simulink model "simu_4qc_transform"  (R2020a)
settings: Solver=FixedStepAuto  StartTime=0.0  StopTime=40  FixedStep=0.01  RelTol=1e-3
InitFcn:
  | init_conditions
values from neighbouring files (symbols this model uses):
  dgaina = 4e-5    (= 4e-05)    [init_conditions.m]
  dgainb = dgaina    (= 4e-05)    [init_conditions.m]
  fd0 = [0;0;m*g/4;0;0;m*g/4;0;0;m*g/4;0;0;m*g/4]    [init_conditions.m]
  g = 9.81    [init_conditions.m]
  IB = diag([IBxy, IBxy, IBz])    [init_conditions.m]
  igaina = 0e-5    (= 0)    [init_conditions.m]
  igainb = igaina    (= 0)    [init_conditions.m]
  Lh = 0.001    [init_conditions.m]
  Lw = 0.18    [init_conditions.m]
  m = (m_qc+0.006)*4 + m_main    (= 0.156)    [init_conditions.m]
  m_main = 0.012    [init_conditions.m]
  m_qc = 0.03    [init_conditions.m]
  np = [np1; np2; np3; np4; np5; ones(numpad,1)*np5(end,:)]    [init_conditions.m]
  pgaina = 1.5e-4    (= 0.00015)    [init_conditions.m]
  pgainb = pgaina    (= 0.00015)    [init_conditions.m]
  phi = zeros(num1+num2+num3+num4+num5+numpad, 1)    [init_conditions.m]
  psi = zeros(num1+num2+num3+num4+num5+numpad, 1)    [init_conditions.m]
  StepSize = 0.01    [init_conditions.m]
  the = [zeros(1,num1+num2), th, th(end) * ones(1, num4+num5+numpad)].'    [init_conditions.m]
undefined symbols (not defined in the file or in its folder): X, Y, Z
libraries: sm_lib x51, nesl_utility x26, simulink_extras x12, simulink x8, sharedtransform x1
(part 1 of 2)
settings Model: Creator=Paul  LastModifiedBy=Paul
settings DataIOCC: ReturnWorkspaceOutputs=off
settings DebuggingCC: ArithmeticOperatorsInVariantConditions=warning
settings SFSimCC: SimUseLocalCustomCode=off  CustomCodeUndefinedFunction=UseInterfaceOnly
settings RTWCC: RTWUseLocalCustomCode=off

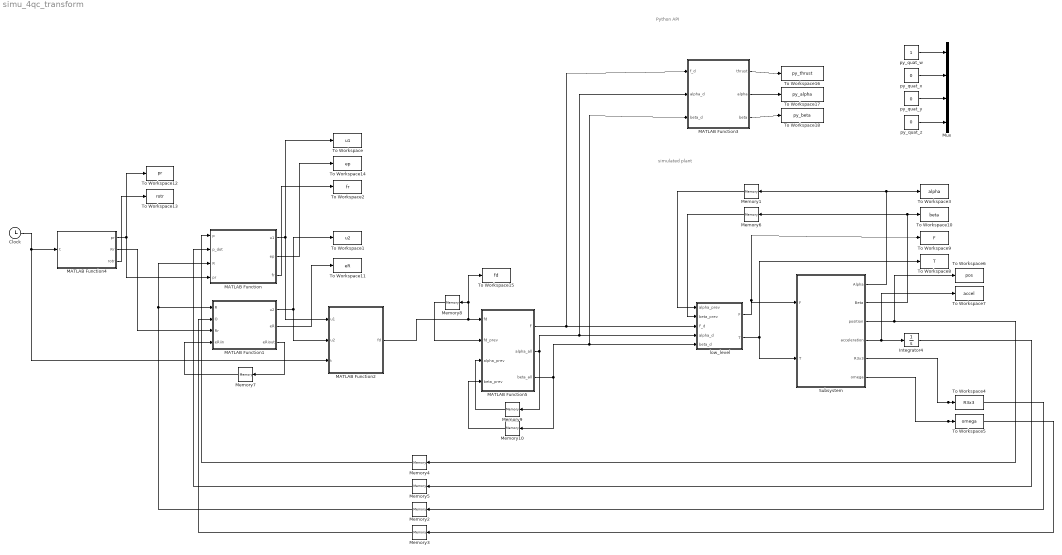
== system simu_4qc_transform ==
  note: Python API
  note: simulated plant
  Clock : Clock
  Integrator4 : Integrator  InitialCondition=[0;0;0]
  MATLAB Function : MATLAB Function  TreatAsAtomicUnit=on
  MATLAB Function1 : MATLAB Function  TreatAsAtomicUnit=on
  MATLAB Function2 : MATLAB Function  TreatAsAtomicUnit=on
  MATLAB Function3 : MATLAB Function  TreatAsAtomicUnit=on
  MATLAB Function4 : MATLAB Function  TreatAsAtomicUnit=on
  MATLAB Function5 : MATLAB Function  TreatAsAtomicUnit=on
  Memory{1,6,9..10} (4 alike) : Memory  InitialCondition=[0;0;0;0]
  Memory2 : Memory  InitialCondition=eye(3)
  Memory{3..5,7} (4 alike) : Memory  InitialCondition=[0;0;0]
  Memory8 : Memory  InitialCondition=fd0
  Mux : Mux
  Subsystem : Subsystem
  To Workspace : ToWorkspace  VariableName=u1  SaveFormat=Timeseries  SampleTime=-1
  To Workspace1 : ToWorkspace  VariableName=u2  SaveFormat=Timeseries  SampleTime=-1
  To Workspace10 : ToWorkspace  VariableName=beta  SaveFormat=Timeseries  SampleTime=-1
  To Workspace11 : ToWorkspace  VariableName=eR  SaveFormat=Timeseries  SampleTime=-1
  To Workspace12 : ToWorkspace  VariableName=pr  SaveFormat=Timeseries  SampleTime=-1
  To Workspace13 : ToWorkspace  VariableName=rotr  SaveFormat=Timeseries  SampleTime=-1
  To Workspace14 : ToWorkspace  VariableName=ep  SaveFormat=Timeseries  SampleTime=-1
  To Workspace15 : ToWorkspace  VariableName=fd  SaveFormat=Timeseries  SampleTime=-1
  To Workspace16 : ToWorkspace  VariableName=py_thrust  SampleTime=-1
      settings: Save2DSignal=2-D array (concatenate along first dimension)
  To Workspace17 : ToWorkspace  VariableName=py_alpha  SampleTime=-1
      settings: Save2DSignal=2-D array (concatenate along first dimension)
  To Workspace18 : ToWorkspace  VariableName=py_beta  SampleTime=-1
      settings: Save2DSignal=2-D array (concatenate along first dimension)
  To Workspace2 : ToWorkspace  VariableName=fr  SaveFormat=Timeseries  SampleTime=-1
  To Workspace3 : ToWorkspace  VariableName=alpha  SaveFormat=Timeseries  SampleTime=-1
  To Workspace4 : ToWorkspace  VariableName=R3x3  SaveFormat=Timeseries  SampleTime=-1
  To Workspace5 : ToWorkspace  VariableName=omega  SaveFormat=Timeseries  SampleTime=-1
  To Workspace6 : ToWorkspace  VariableName=pos  SaveFormat=Timeseries  SampleTime=-1
  To Workspace7 : ToWorkspace  VariableName=accel  SaveFormat=Timeseries  SampleTime=-1
  To Workspace8 : ToWorkspace  VariableName=T  SaveFormat=Timeseries  SampleTime=-1
  To Workspace9 : ToWorkspace  VariableName=F  SaveFormat=Timeseries  SampleTime=-1
  low_level : Subsystem
  py_quat_w : Constant
  py_quat_x : Constant  Value=0
  py_quat_y : Constant  Value=0
  py_quat_z : Constant  Value=0
  wires:
  MATLAB Function/1(u1) -> MATLAB Function2/1(u1), To Workspace/1
  MATLAB Function1/1(u2) -> MATLAB Function2/2(u2), To Workspace1/1
  Subsystem/5(R3x3) -> To Workspace4/1, Memory2/1
  Memory2/1 -> MATLAB Function1/1(R), MATLAB Function/3(R)
  Subsystem/6(omega) -> To Workspace5/1, Memory3/1
  Memory3/1 -> MATLAB Function1/2(O)
  Memory4/1 -> MATLAB Function/1(p)
  Memory5/1 -> MATLAB Function/2(p_dot)
  Subsystem/3(position) -> Memory4/1, To Workspace6/1
  Subsystem/4(acceleration) -> Integrator4/1, To Workspace7/1
  Integrator4/1 -> Memory5/1
  Clock/1 -> MATLAB Function2/3(t), MATLAB Function4/1(t)
  MATLAB Function4/1(pr) -> MATLAB Function/4(pr), To Workspace12/1
  MATLAB Function4/2(Rr) -> MATLAB Function1/3(Rr)
  MATLAB Function/3(fr) -> To Workspace2/1
  low_level/1(F) -> To Workspace9/1, Subsystem/1(F)
  low_level/2(T) -> To Workspace8/1, Subsystem/2(T)
  Subsystem/1(Alpha) -> To Workspace3/1, Memory1/1
  Subsystem/2(Beta) -> Memory6/1, To Workspace10/1
  Memory1/1 -> low_level/1(alpha_prev)
  Memory6/1 -> low_level/2(beta_prev)
  MATLAB Function1/2(eR) -> To Workspace11/1
  MATLAB Function4/3(rotr) -> To Workspace13/1
  MATLAB Function/2(ep) -> To Workspace14/1
  MATLAB Function1/3(eRiout) -> Memory7/1
  Memory7/1 -> MATLAB Function1/4(eRiin)
  Memory10/1 -> MATLAB Function5/4(beta_prev)
  Memory8/1 -> MATLAB Function5/2(fd_prev)
  MATLAB Function5/3(beta_all) -> MATLAB Function3/3(beta_d), low_level/5(beta_d), Memory10/1
  MATLAB Function5/2(alpha_all) -> MATLAB Function3/2(alpha_d), low_level/4(alpha_d), Memory9/1
  Memory9/1 -> MATLAB Function5/3(alpha_prev)
  MATLAB Function2/1(fd) -> To Workspace15/1, Memory8/1, MATLAB Function5/1(fd)
  MATLAB Function5/1(F) -> MATLAB Function3/1(f_d), low_level/3(F_d)
  MATLAB Function3/1(thrust) -> To Workspace16/1
  MATLAB Function3/2(alpha) -> To Workspace17/1
  MATLAB Function3/3(beta) -> To Workspace18/1
  py_quat_w/1 -> Mux/1
  py_quat_x/1 -> Mux/2
  py_quat_y/1 -> Mux/3
  py_quat_z/1 -> Mux/4

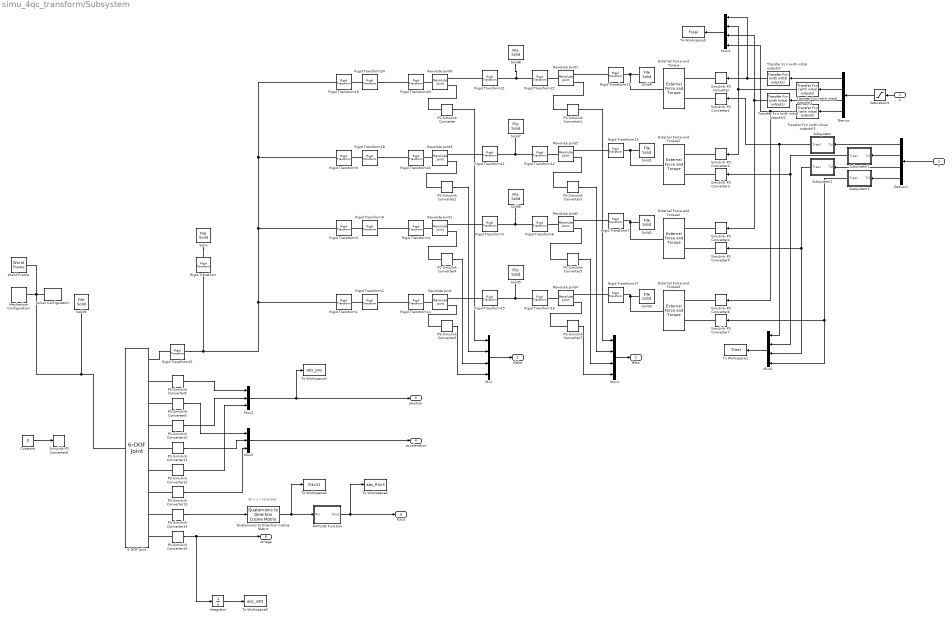
== system simu_4qc_transform/Subsystem ==
  note: all x y z reversed
  F : Inport
  T : Inport  Port=2
  6-DOF Joint : sm_lib/Joints/6-DOF Joint  JointMode=Normal  SenseConstraintForce=off  SenseConstraintForceX=off  SenseConstraintForceY=off  SenseConstraintForceZ=off  SenseConstraintTorque=off  SenseConstraintTorqueX=off  SenseConstraintTorqueY=off  SenseConstraintTorqueZ=off  SenseTotalForce=off  SenseTotalForceX=off  SenseTotalForceY=off  SenseTotalForceZ=off  SenseTotalTorque=off  SenseTotalTorqueX=off  SenseTotalTorqueY=off  SenseTotalTorqueZ=off  CompositeWrenchDir=FollowerOnBase  CompositeWrenchFrame=BaseFrame  PxEquilibriumPosition=0  PxEquilibriumPositionUnits=m  PxSpringStiffness=0  PxSpringStiffnessUnits=N/m  PxDampingCoefficient=0  PxDampingCoefficientUnits=N/(m/s)  PxTorqueActuationMode=NoTorque  PxMotionActuationMode=ComputedMotion  PxSensePosition=on  PxSenseVelocity=off  PxSenseAcceleration=on  PxSenseTorqueForce=off  PxSenseLowerLimitTorqueForce=off  PxSenseUpperLimitTorqueForce=off  PxLowerLimitSpecify=off  PxLowerLimitBound=-1  PxLowerLimitBoundUnits=m  PxLowerLimitStiffness=1e6  PxLowerLimitStiffnessUnits=N/m  PxLowerLimitDamping=1e3  PxLowerLimitDampingUnits=N/(m/s)  PxLowerLimitTransitionRegionWidth=1e-4  PxLowerLimitTransitionRegionWidthUnits=m  PxUpperLimitSpecify=off  PxUpperLimitBound=1  PxUpperLimitBoundUnits=m  PxUpperLimitStiffness=1e6  PxUpperLimitStiffnessUnits=N/m  PxUpperLimitDamping=1e3  PxUpperLimitDampingUnits=N/(m/s)  PxUpperLimitTransitionRegionWidth=1e-4  PxUpperLimitTransitionRegionWidthUnits=m  PxPositionTargetSpecify=off  PxPositionTargetPriority=High  PxPositionTargetValue=0  PxPositionTargetValueUnits=m  PxVelocityTargetSpecify=off  PxVelocityTargetPriority=High  PxVelocityTargetValue=0  PxVelocityTargetValueUnits=m/s  PyEquilibriumPosition=0  PyEquilibriumPositionUnits=m  PySpringStiffness=0  PySpringStiffnessUnits=N/m  PyDampingCoefficient=0  PyDampingCoefficientUnits=N/(m/s)  PyTorqueActuationMode=NoTorque  PyMotionActuationMode=ComputedMotion  PySensePosition=on  PySenseVelocity=off  PySenseAcceleration=on  PySenseTorqueForce=off  PySenseLowerLimitTorqueForce=off  PySenseUpperLimitTorqueForce=off  PyLowerLimitSpecify=off  PyLowerLimitBound=-1  PyLowerLimitBoundUnits=m  PyLowerLimitStiffness=1e6  PyLowerLimitStiffnessUnits=N/m  PyLowerLimitDamping=1e3  PyLowerLimitDampingUnits=N/(m/s)  PyLowerLimitTransitionRegionWidth=1e-4  PyLowerLimitTransitionRegionWidthUnits=m  PyUpperLimitSpecify=off  PyUpperLimitBound=1  PyUpperLimitBoundUnits=m  PyUpperLimitStiffness=1e6  PyUpperLimitStiffnessUnits=N/m  PyUpperLimitDamping=1e3  PyUpperLimitDampingUnits=N/(m/s)  PyUpperLimitTransitionRegionWidth=1e-4  PyUpperLimitTransitionRegionWidthUnits=m  PyPositionTargetSpecify=off  PyPositionTargetPriority=High  PyPositionTargetValue=0  PyPositionTargetValueUnits=m  PyVelocityTargetSpecify=off  PyVelocityTargetPriority=High  PyVelocityTargetValue=0  PyVelocityTargetValueUnits=m/s  PzEquilibriumPosition=0  PzEquilibriumPositionUnits=m  PzSpringStiffness=0  PzSpringStiffnessUnits=N/m  PzDampingCoefficient=0  PzDampingCoefficientUnits=N/(m/s)  PzTorqueActuationMode=NoTorque  PzMotionActuationMode=ComputedMotion  PzSensePosition=on  PzSenseVelocity=off  PzSenseAcceleration=on  PzSenseTorqueForce=off  PzSenseLowerLimitTorqueForce=off  PzSenseUpperLimitTorqueForce=off  PzLowerLimitSpecify=off  PzLowerLimitBound=-1  PzLowerLimitBoundUnits=m  PzLowerLimitStiffness=1e6  PzLowerLimitStiffnessUnits=N/m  PzLowerLimitDamping=1e3  PzLowerLimitDampingUnits=N/(m/s)  PzLowerLimitTransitionRegionWidth=1e-4  PzLowerLimitTransitionRegionWidthUnits=m  PzUpperLimitSpecify=off  PzUpperLimitBound=1  PzUpperLimitBoundUnits=m  PzUpperLimitStiffness=1e6  PzUpperLimitStiffnessUnits=N/m  PzUpperLimitDamping=1e3  PzUpperLimitDampingUnits=N/(m/s)  PzUpperLimitTransitionRegionWidth=1e-4  PzUpperLimitTransitionRegionWidthUnits=m  PzPositionTargetSpecify=off  PzPositionTargetPriority=High  PzPositionTargetValue=0  PzPositionTargetValueUnits=m  PzVelocityTargetSpecify=off  PzVelocityTargetPriority=High  PzVelocityTargetValue=0  PzVelocityTargetValueUnits=m/s  SphDefPosRotationMethod=None  SphDefPosRotationAngleUnits=deg  SphDefPosRotationStandardAxis=+Z  SphDefPosRotationAngle=0.0  SphDefPosRotationArbitraryAxis=[0 0 1]  SphDefPosFollAlignAxisA=+X  SphDefPosBaseAlignAxisA=+Y  SphDefPosFollAlignAxisB=+Y  SphDefPosBaseAlignAxisB=+Z  SphDefPosRotationSequenceAxes=FollowerAxes  SphDefPosRotationSequence=XYX  SphDefPosRotationSequenceAngles=[0 0 0]  SphDefPosRotationSequenceAnglesUnits=deg  SphDefPosRotationMatrix=[1 0 0; 0 1 0; 0 0 1]  SphEqPosRotationMethod=None  SphEqPosRotationAngleUnits=deg  SphEqPosRotationStandardAxis=+Z  SphEqPosRotationAngle=0.0  SphEqPosRotationArbitraryAxis=[0 0 1]  SphEqPosFollAlignAxisA=+X  SphEqPosBaseAlignAxisA=+Y  SphEqPosFollAlignAxisB=+Y  SphEqPosBaseAlignAxisB=+Z  SphEqPosRotationSequenceAxes=FollowerAxes  SphEqPosRotationSequence=XYX  SphEqPosRotationSequenceAngles=[0 0 0]  SphEqPosRotationSequenceAnglesUnits=deg  SphEqPosRotationMatrix=[1 0 0; 0 1 0; 0 0 1]  SphSpringStiffness=0  SphSpringStiffnessUnits=N*m/deg  SphDampingCoefficient=0  SphDampingCoefficientUnits=N*m/(deg/s)  SphActuateTorqueX=off  SphActuateTorqueY=off  SphActuateTorqueZ=off  SphActuateTorque=off  SphTorqueActuationMode=NoTorque  SphMotionActuationMode=ComputedMotion  SphActuationFrame=BaseFrame  SphSensePosition=on  SphSenseVelocityX=off  SphSenseVelocityY=off  SphSenseVelocityZ=off  SphSenseVelocity=on  SphSenseAccelerationX=off  SphSenseAccelerationY=off  SphSenseAccelerationZ=off  SphSenseAcceleration=off  SphSenseTorqueX=off  SphSenseTorqueY=off  SphSenseTorqueZ=off  SphSenseTorqueForce=off  SphSenseLowerLimitTorqueMag=off  SphSenseUpperLimitTorqueMag=off  SphSensingFrame=BaseFrame  SphLowerLimitSpecify=off  SphLowerLimitBound=15  SphLowerLimitBoundUnits=deg  SphLowerLimitStiffness=1e4  SphLowerLimitStiffnessUnits=N*m/deg  SphLowerLimitDamping=10  SphLowerLimitDampingUnits=N*m/(deg/s)  SphLowerLimitTransitionRegionWidth=0.1  SphLowerLimitTransitionRegionWidthUnits=deg  SphUpperLimitSpecify=off  SphUpperLimitBound=45  SphUpperLimitBoundUnits=deg  SphUpperLimitStiffness=1e4  SphUpperLimitStiffnessUnits=N*m/deg  SphUpperLimitDamping=10  SphUpperLimitDampingUnits=N*m/(deg/s)  SphUpperLimitTransitionRegionWidth=0.1  SphUpperLimitTransitionRegionWidthUnits=deg  SphPositionTargetRotationMethod=None  SphPositionTargetRotationAngleUnits=deg  SphPositionTargetRotationStandardAxis=+Z  SphPositionTargetRotationAngle=0.0  SphPositionTargetRotationArbitraryAxis=[0 0 1]  SphPositionTargetFollAlignAxisA=+X  SphPositionTargetBaseAlignAxisA=+Y  SphPositionTargetFollAlignAxisB=+Y  SphPositionTargetBaseAlignAxisB=+Z  SphPositionTargetRotationSequenceAxes=FollowerAxes  SphPositionTargetRotationSequence=XYX  SphPositionTargetRotationSequenceAngles=[0 0 0]  SphPositionTargetRotationSequenceAnglesUnits=deg  SphPositionTargetRotationMatrix=[1 0 0; 0 1 0; 0 0 1]  SphPositionTargetSpecify=off  SphPositionTargetPriority=High  SphVelocityTargetValue=[0 0 0]  SphVelocityTargetValueUnits=deg/s  SphVelocityTargetSpecify=off  SphVelocityTargetPriority=High  SphVelocityTargetInFollowerFrame=on
  Constant : Constant  Value=0
  Demux : Demux
  Demux1 : Demux
  External Force and Torque{,1..3} (4 alike) : sm_lib/Forces and Torques/External Force and Torque  ForceResolutionFrame=AttachedFrame  EnableForceX=off  EnableForceY=off  EnableForceZ=on  EnableForce=off  TorqueResolutionFrame=AttachedFrame  EnableTorqueX=off  EnableTorqueY=off  EnableTorqueZ=off  EnableTorque=on
  Integrator : Integrator
  MATLAB Function : MATLAB Function  TreatAsAtomicUnit=on
  Mechanism Configuration : sm_lib/Utilities/Mechanism Configuration  UniformGravity=Constant  GravityVector=[0 0 -9.81]  GravityUnits=m/s^2  LinearizationDelta=0.002
  Mux{,1,4..5} (4 alike) : Mux
  Mux2 : Mux  Inputs=3
  Mux3 : Mux  Inputs=3
  PS-Simulink Converter{,1..15} (16 alike) : nesl_utility/PS-Simulink Converter  PhysicalDomain=network_engine_domain  SubClassName=ps_output  LeftPortType=input  RightPortType=output  PseudoPeriodic=off  Frequencies=[]  Unit=1  AffineConversion=off
  Quaternions to Direction Cosine Matrix : sharedtransform/Quaternions to  Direction Cosine Matrix  aMode=aMode
      settings: SourceProductBaseCode=AE,PW,MT,VE,VP
  Revolute Joint{,1..7} (8 alike) : sm_lib/Joints/Revolute Joint  JointMode=Normal  SenseConstraintForce=off  SenseConstraintForceX=off  SenseConstraintForceY=off  SenseConstraintForceZ=off  SenseConstraintTorque=off  SenseConstraintTorqueX=off  SenseConstraintTorqueY=off  SenseConstraintTorqueZ=off  SenseTotalForce=off  SenseTotalForceX=off  SenseTotalForceY=off  SenseTotalForceZ=off  SenseTotalTorque=off  SenseTotalTorqueX=off  SenseTotalTorqueY=off  SenseTotalTorqueZ=off  CompositeWrenchDir=FollowerOnBase  CompositeWrenchFrame=BaseFrame  EquilibriumPosition=0  EquilibriumPositionUnits=deg  SpringStiffness=0  SpringStiffnessUnits=N*m/deg  DampingCoefficient=0  DampingCoefficientUnits=N*m/(deg/s)  TorqueActuationMode=NoTorque  MotionActuationMode=ComputedMotion  SensePosition=on  SenseVelocity=off  SenseAcceleration=off  SenseTorqueForce=off  SenseLowerLimitTorqueForce=off  SenseUpperLimitTorqueForce=off  LowerLimitSpecify=off  LowerLimitBound=-90  LowerLimitBoundUnits=deg  LowerLimitStiffness=1e4  LowerLimitStiffnessUnits=N*m/deg  LowerLimitDamping=10  LowerLimitDampingUnits=N*m/(deg/s)  LowerLimitTransitionRegionWidth=0.1  LowerLimitTransitionRegionWidthUnits=deg  UpperLimitSpecify=off  UpperLimitBound=90  UpperLimitBoundUnits=deg  UpperLimitStiffness=1e4  UpperLimitStiffnessUnits=N*m/deg  UpperLimitDamping=10  UpperLimitDampingUnits=N*m/(deg/s)  UpperLimitTransitionRegionWidth=0.1  UpperLimitTransitionRegionWidthUnits=deg  PositionTargetSpecify=off  PositionTargetPriority=High  PositionTargetValue=0  PositionTargetValueUnits=deg  VelocityTargetSpecify=off  VelocityTargetPriority=High  VelocityTargetValue=0  VelocityTargetValueUnits=deg/s
  Rigid Transform : sm_lib/Frames and Transforms/Rigid Transform  TranslationMethod=None  TranslationStandardOffset=0  TranslationLengthUnit=m  TranslationStandardAxis=+Z  TranslationCartesianOffset=[0 0 0]  TranslationROffset=0  TranslationROffsetUnits=m  TranslationZOffset=0  TranslationZOffsetUnits=m  TranslationThetaOffset=0  TranslationThetaOffsetUnits=deg  RotationMethod=None  RotationAngleUnits=deg  RotationStandardAxis=+Z  RotationAngle=0.0  RotationArbitraryAxis=[0 0 1]  FollAlignAxisA=+X  BaseAlignAxisA=+Y  FollAlignAxisB=+Y  BaseAlignAxisB=+Z  RotationSequenceAxes=FollowerAxes  RotationSequence=XYX  RotationSequenceAngles=[0 0 0]  RotationSequenceAnglesUnits=deg  RotationMatrix=[1 0 0; 0 1 0; 0 0 1]
  Rigid Transform1 : sm_lib/Frames and Transforms/Rigid Transform  TranslationMethod=None  TranslationStandardOffset=0  TranslationLengthUnit=m  TranslationStandardAxis=+Z  TranslationCartesianOffset=[0 0 0]  TranslationROffset=0  TranslationROffsetUnits=m  TranslationZOffset=0  TranslationZOffsetUnits=m  TranslationThetaOffset=0  TranslationThetaOffsetUnits=deg  RotationMethod=StandardAxis  RotationAngleUnits=deg  RotationStandardAxis=+Z  RotationAngle=270  RotationArbitraryAxis=[0 0 1]  FollAlignAxisA=+X  BaseAlignAxisA=+Y  FollAlignAxisB=+Y  BaseAlignAxisB=+Z  RotationSequenceAxes=FollowerAxes  RotationSequence=XYX  RotationSequenceAngles=[0 0 0]  RotationSequenceAnglesUnits=deg  RotationMatrix=[1 0 0; 0 1 0; 0 0 1]
  Rigid Transform{4,10,14,20} (4 alike) : sm_lib/Frames and Transforms/Rigid Transform  TranslationMethod=None  TranslationStandardOffset=0.4  TranslationLengthUnit=m  TranslationStandardAxis=+X  TranslationCartesianOffset=[0 0 0]  TranslationROffset=0  TranslationROffsetUnits=m  TranslationZOffset=0  TranslationZOffsetUnits=m  TranslationThetaOffset=0  TranslationThetaOffsetUnits=deg  RotationMethod=StandardAxis  RotationAngleUnits=deg  RotationStandardAxis=+Y  RotationAngle=90  RotationArbitraryAxis=[0 0 1]  FollAlignAxisA=+X  BaseAlignAxisA=+Y  FollAlignAxisB=+Y  BaseAlignAxisB=+Z  RotationSequenceAxes=FollowerAxes  RotationSequence=XYX  RotationSequenceAngles=[0 0 0]  RotationSequenceAnglesUnits=deg  RotationMatrix=[1 0 0; 0 1 0; 0 0 1]
  Rigid Transform{5,11,15,21} (4 alike) : sm_lib/Frames and Transforms/Rigid Transform  TranslationMethod=None  TranslationStandardOffset=0.4  TranslationLengthUnit=m  TranslationStandardAxis=+X  TranslationCartesianOffset=[0 0 0]  TranslationROffset=0  TranslationROffsetUnits=m  TranslationZOffset=0  TranslationZOffsetUnits=m  TranslationThetaOffset=0  TranslationThetaOffsetUnits=deg  RotationMethod=StandardAxis  RotationAngleUnits=deg  RotationStandardAxis=-Y  RotationAngle=90  RotationArbitraryAxis=[0 0 1]  FollAlignAxisA=+X  BaseAlignAxisA=+Y  FollAlignAxisB=+Y  BaseAlignAxisB=+Z  RotationSequenceAxes=FollowerAxes  RotationSequence=XYX  RotationSequenceAngles=[0 0 0]  RotationSequenceAnglesUnits=deg  RotationMatrix=[1 0 0; 0 1 0; 0 0 1]
  Rigid Transform{6,12,16,22} (4 alike) : sm_lib/Frames and Transforms/Rigid Transform  TranslationMethod=None  TranslationStandardOffset=0.4  TranslationLengthUnit=m  TranslationStandardAxis=+X  TranslationCartesianOffset=[0 0 0]  TranslationROffset=0  TranslationROffsetUnits=m  TranslationZOffset=0  TranslationZOffsetUnits=m  TranslationThetaOffset=0  TranslationThetaOffsetUnits=deg  RotationMethod=StandardAxis  RotationAngleUnits=deg  RotationStandardAxis=-X  RotationAngle=90  RotationArbitraryAxis=[0 0 1]  FollAlignAxisA=+X  BaseAlignAxisA=+Y  FollAlignAxisB=+Y  BaseAlignAxisB=+Z  RotationSequenceAxes=FollowerAxes  RotationSequence=XYX  RotationSequenceAngles=[0 0 0]  RotationSequenceAnglesUnits=deg  RotationMatrix=[1 0 0; 0 1 0; 0 0 1]
  Rigid Transform{7,13,17,23} (4 alike) : sm_lib/Frames and Transforms/Rigid Transform  TranslationMethod=None  TranslationStandardOffset=0.4  TranslationLengthUnit=m  TranslationStandardAxis=+X  TranslationCartesianOffset=[0 0 0]  TranslationROffset=0  TranslationROffsetUnits=m  TranslationZOffset=0  TranslationZOffsetUnits=m  TranslationThetaOffset=0  TranslationThetaOffsetUnits=deg  RotationMethod=StandardAxis  RotationAngleUnits=deg  RotationStandardAxis=+X  RotationAngle=90  RotationArbitraryAxis=[0 0 1]  FollAlignAxisA=+X  BaseAlignAxisA=+Y  FollAlignAxisB=+Y  BaseAlignAxisB=+Z  RotationSequenceAxes=FollowerAxes  RotationSequence=XYX  RotationSequenceAngles=[0 0 0]  RotationSequenceAnglesUnits=deg  RotationMatrix=[1 0 0; 0 1 0; 0 0 1]
  Rigid Transform{2,8,18,24} (4 alike) : sm_lib/Frames and Transforms/Rigid Transform  TranslationMethod=StandardAxis  TranslationStandardOffset=0.18  TranslationLengthUnit=m  TranslationStandardAxis=+X  TranslationCartesianOffset=[0 0 0]  TranslationROffset=0  TranslationROffsetUnits=m  TranslationZOffset=0  TranslationZOffsetUnits=m  TranslationThetaOffset=0  TranslationThetaOffsetUnits=deg  RotationMethod=None  RotationAngleUnits=deg  RotationStandardAxis=+Z  RotationAngle=0.0  RotationArbitraryAxis=[0 0 1]  FollAlignAxisA=+X  BaseAlignAxisA=+Y  FollAlignAxisB=+Y  BaseAlignAxisB=+Z  RotationSequenceAxes=FollowerAxes  RotationSequence=XYX  RotationSequenceAngles=[0 0 0]  RotationSequenceAnglesUnits=deg  RotationMatrix=[1 0 0; 0 1 0; 0 0 1]
  Rigid Transform19 : sm_lib/Frames and Transforms/Rigid Transform  TranslationMethod=None  TranslationStandardOffset=0  TranslationLengthUnit=m  TranslationStandardAxis=+Z  TranslationCartesianOffset=[0 0 0]  TranslationROffset=0  TranslationROffsetUnits=m  TranslationZOffset=0  TranslationZOffsetUnits=m  TranslationThetaOffset=0  TranslationThetaOffsetUnits=deg  RotationMethod=StandardAxis  RotationAngleUnits=deg  RotationStandardAxis=+Z  RotationAngle=0  RotationArbitraryAxis=[0 0 1]  FollAlignAxisA=+X  BaseAlignAxisA=+Y  FollAlignAxisB=+Y  BaseAlignAxisB=+Z  RotationSequenceAxes=FollowerAxes  RotationSequence=XYX  RotationSequenceAngles=[0 0 0]  RotationSequenceAnglesUnits=deg  RotationMatrix=[1 0 0; 0 1 0; 0 0 1]
  Rigid Transform25 : sm_lib/Frames and Transforms/Rigid Transform  TranslationMethod=StandardAxis  TranslationStandardOffset=Lh  TranslationLengthUnit=m  TranslationStandardAxis=-Z  TranslationCartesianOffset=[0 0 0]  TranslationROffset=0  TranslationROffsetUnits=m  TranslationZOffset=0  TranslationZOffsetUnits=m  TranslationThetaOffset=0  TranslationThetaOffsetUnits=deg  RotationMethod=None  RotationAngleUnits=deg  RotationStandardAxis=+Z  RotationAngle=270  RotationArbitraryAxis=[0 0 1]  FollAlignAxisA=+X  BaseAlignAxisA=+Y  FollAlignAxisB=+Y  BaseAlignAxisB=+Z  RotationSequenceAxes=FollowerAxes  RotationSequence=XYX  RotationSequenceAngles=[0 0 0]  RotationSequenceAnglesUnits=deg  RotationMatrix=[1 0 0; 0 1 0; 0 0 1]
  Rigid Transform3 : sm_lib/Frames and Transforms/Rigid Transform  TranslationMethod=None  TranslationStandardOffset=0  TranslationLengthUnit=m  TranslationStandardAxis=+Z  TranslationCartesianOffset=[0 0 0]  TranslationROffset=0  TranslationROffsetUnits=m  TranslationZOffset=0  TranslationZOffsetUnits=m  TranslationThetaOffset=0  TranslationThetaOffsetUnits=deg  RotationMethod=StandardAxis  RotationAngleUnits=deg  RotationStandardAxis=+Z  RotationAngle=180  RotationArbitraryAxis=[0 0 1]  FollAlignAxisA=+X  BaseAlignAxisA=+Y  FollAlignAxisB=+Y  BaseAlignAxisB=+Z  RotationSequenceAxes=FollowerAxes  RotationSequence=XYX  RotationSequenceAngles=[0 0 0]  RotationSequenceAnglesUnits=deg  RotationMatrix=[1 0 0; 0 1 0; 0 0 1]
  Rigid Transform9 : sm_lib/Frames and Transforms/Rigid Transform  TranslationMethod=None  TranslationStandardOffset=0  TranslationLengthUnit=m  TranslationStandardAxis=+Z  TranslationCartesianOffset=[0 0 0]  TranslationROffset=0  TranslationROffsetUnits=m  TranslationZOffset=0  TranslationZOffsetUnits=m  TranslationThetaOffset=0  TranslationThetaOffsetUnits=deg  RotationMethod=StandardAxis  RotationAngleUnits=deg  RotationStandardAxis=+Z  RotationAngle=90  RotationArbitraryAxis=[0 0 1]  FollAlignAxisA=+X  BaseAlignAxisA=+Y  FollAlignAxisB=+Y  BaseAlignAxisB=+Z  RotationSequenceAxes=FollowerAxes  RotationSequence=XYX  RotationSequenceAngles=[0 0 0]  RotationSequenceAnglesUnits=deg  RotationMatrix=[1 0 0; 0 1 0; 0 0 1]
  Saturation3 : Saturate  UpperLimit=0.5886  LowerLimit=0
  Simulink-PS Converter{,1..8} (9 alike) : nesl_utility/Simulink-PS Converter  PhysicalDomain=network_engine_domain  SubClassName=ps_input  LeftPortType=input  RightPortType=output  PseudoPeriodic=off  Frequencies=[]  NoiseDistribution=none  NoiseParameters=[]  Unit=1  AffineConversion=off  FilteringAndDerivatives=provide  SimscapeFilterOrder=1  InputFilterTimeConstant=0.001  UdotUserProvided=0
  Solid : sm_lib/Body Elements/File Solid  ExtGeomFileName=.\main_frame.STEP  UnitType=FromFile  ExtGeomFileUnits=m  StepReaderType=HEX  ExportConvexHullGeometry=off  InertiaType=Custom  Mass=m_main  MassUnits=kg  CenterOfMass=[0 0 0]  CenterOfMassUnits=m  MomentsOfInertia=[3e-5 3e-5 6e-5]  MomentsOfInertiaUnits=kg*m^2  ProductsOfInertia=[0 0 0]  ProductsOfInertiaUnits=kg*m^2  BasedOnType=Density  Density=1000  DensityUnits=kg/m^3  DoExposeReferenceFrame=on  SerializedFrames=<Frames/>  GraphicType=FromGeometry  MarkerShape=Sphere  MarkerSize=10  GraphicVisPropType=SimpleVisualProperties  GraphicDiffuseColor=[0.2 0.2 0.2]  GraphicSpecularColor=[0.5 0.5 0.5 1.0]  GraphicAmbientColor=[0.15 0.15 0.15 1.0]  GraphicEmissiveColor=[0.0 0.0 0.0 1.0]  GraphicShininess=75  GraphicOpacity=1.0
  Solid{1..4} (4 alike) : sm_lib/Body Elements/File Solid  ExtGeomFileName=.\qcscheme.STEP  UnitType=FromFile  ExtGeomFileUnits=m  StepReaderType=HEX  ExportConvexHullGeometry=off  InertiaType=Custom  Mass=m_qc  MassUnits=kg  CenterOfMass=[0 0 0]  CenterOfMassUnits=m  MomentsOfInertia=[1.2e-5 1.2e-5 2.2e-5]  MomentsOfInertiaUnits=kg*m^2  ProductsOfInertia=[0 0 0]  ProductsOfInertiaUnits=kg*m^2  BasedOnType=Density  Density=1000  DensityUnits=kg/m^3  DoExposeReferenceFrame=on  SerializedFrames=<Frames/>  GraphicType=FromGeometry  MarkerShape=Sphere  MarkerSize=10  GraphicVisPropType=SimpleVisualProperties  GraphicDiffuseColor=[0.5 0.5 0.5]  GraphicSpecularColor=[0.5 0.5 0.5 1.0]  GraphicAmbientColor=[0.15 0.15 0.15 1.0]  GraphicEmissiveColor=[0.0 0.0 0.0 1.0]  GraphicShininess=75  GraphicOpacity=1.0
  Solid{5..8} (4 alike) : sm_lib/Body Elements/File Solid  ExtGeomFileName=.\ring.STEP  UnitType=FromFile  ExtGeomFileUnits=m  StepReaderType=HEX  ExportConvexHullGeometry=off  InertiaType=Custom  Mass=0.006  MassUnits=kg  CenterOfMass=[0 0 0]  CenterOfMassUnits=m  MomentsOfInertia=[1e-6 1e-6 1e-6]  MomentsOfInertiaUnits=kg*m^2  ProductsOfInertia=[0 0 0]  ProductsOfInertiaUnits=kg*m^2  BasedOnType=Density  Density=1000  DensityUnits=kg/m^3  DoExposeReferenceFrame=on  SerializedFrames=<Frames/>  GraphicType=FromGeometry  MarkerShape=Sphere  MarkerSize=10  GraphicVisPropType=SimpleVisualProperties  GraphicDiffuseColor=[1.0 0.6 0.0]  GraphicSpecularColor=[0.5 0.5 0.5 1.0]  GraphicAmbientColor=[0.15 0.15 0.15 1.0]  GraphicEmissiveColor=[0.0 0.0 0.0 1.0]  GraphicShininess=75  GraphicOpacity=1.0
  Solid9 : sm_lib/Body Elements/File Solid  ExtGeomFileName=.\circle_traj.STEP  UnitType=FromFile  ExtGeomFileUnits=m  StepReaderType=HEX  ExportConvexHullGeometry=off  InertiaType=Custom  Mass=m_main  MassUnits=kg  CenterOfMass=[0 0 0]  CenterOfMassUnits=m  MomentsOfInertia=[3e-5 3e-5 6e-5]  MomentsOfInertiaUnits=kg*m^2  ProductsOfInertia=[0 0 0]  ProductsOfInertiaUnits=kg*m^2  BasedOnType=Density  Density=1000  DensityUnits=kg/m^3  DoExposeReferenceFrame=on  SerializedFrames=<Frames/>  GraphicType=FromGeometry  MarkerShape=Sphere  MarkerSize=10  GraphicVisPropType=SimpleVisualProperties  GraphicDiffuseColor=[0.4 1.0 0.0]  GraphicSpecularColor=[0.5 0.5 0.5 1.0]  GraphicAmbientColor=[0.15 0.15 0.15 1.0]  GraphicEmissiveColor=[0.0 0.0 0.0 1.0]  GraphicShininess=75  GraphicOpacity=1.0
  Solver Configuration : nesl_utility/Solver Configuration  PhysicalDomain=network_engine_domain  SubClassName=solver  LeftPortType=input  RightPortType=generic  Tones=[]  Harmonics=[]  SimulateNoise=off  Profile=off  UseLocalSampling=off  EnableSwitchedLinearOptims=on  FrequencyDomain=off  UseCCode=off  RelTol=0.001  AbsTol=1e-06  MinStep=1e-09  ToWorkspace=off  RevertToSquareIcSolve=off  NumHomotopyIterations=100  PhasorMode=off  PhasorModeNumHarmonics=1  DoDC=off  ResidualTolerance=1e-09  UseLocalSolver=off  LocalSolverChoice=NE_BACKWARD_EULER_ADVANCER  LocalSolverSampleTime=0.001  DoFixedCost=off  MaxNonlinIter=3  MaxModeIter=2  LinearAlgebra=Sparse  EquationFormulation=NE_TIME_EF  DelaysMemoryBudget=1024  AutomaticFiltering=on  FilteringTimeConstant=0.002  PartitionStorageMethod=AS_NEEDED  PartitionMemoryBudget=1024  PartitionMethod=FAST
  Subsystem : Subsystem
  Subsystem1 : Subsystem
  Subsystem2 : Subsystem
  Subsystem3 : Subsystem
  To Workspace1 : ToWorkspace  VariableName=Treal  SaveFormat=Timeseries  SampleTime=-1
  To Workspace2 : ToWorkspace  VariableName=abs_R3x3  SaveFormat=Timeseries  SampleTime=-1
  To Workspace3 : ToWorkspace  VariableName=abs_pos  SaveFormat=Timeseries  SampleTime=-1
  To Workspace4 : ToWorkspace  VariableName=R3x31  SaveFormat=Timeseries  SampleTime=-1
  To Workspace5 : ToWorkspace  VariableName=abs_intO  SaveFormat=Timeseries  SampleTime=-1
  To Workspace9 : ToWorkspace  VariableName=Freal  SaveFormat=Timeseries  SampleTime=-1
  Transfer Fcn (with initial outputs){,1..3} (4 alike) : simulink_extras/Additional Linear/Transfer Fcn (with initial outputs)  N=[1]  D="[0.01  1]"  Y0=m*g/4  U0=m*g/4
  World Frame : sm_lib/Frames and Transforms/World Frame
  Alpha : Outport  VectorParamsAs1DForOutWhenUnconnected=off
  Beta : Outport  Port=2  VectorParamsAs1DForOutWhenUnconnected=off
  position : Outport  Port=3  VectorParamsAs1DForOutWhenUnconnected=off
  acceleration : Outport  Port=4  VectorParamsAs1DForOutWhenUnconnected=off
  R3x3 : Outport  Port=5  VectorParamsAs1DForOutWhenUnconnected=off
  omega : Outport  Port=6  VectorParamsAs1DForOutWhenUnconnected=off
  wires:
  PS-Simulink Converter6/1 -> Mux/4
  PS-Simulink Converter/1 -> Mux/1
  PS-Simulink Converter2/1 -> Mux/2
  PS-Simulink Converter4/1 -> Mux/3
  PS-Simulink Converter1/1 -> Mux1/1
  PS-Simulink Converter7/1 -> Mux1/4
  PS-Simulink Converter3/1 -> Mux1/2
  PS-Simulink Converter5/1 -> Mux1/3
  Mux/1 -> Alpha/1
  Mux1/1 -> Beta/1
  PS-Simulink Converter14/1 -> Quaternions to Direction Cosine Matrix/1
  Quaternions to Direction Cosine Matrix/1 -> To Workspace4/1, MATLAB Function/1(Rin)
  PS-Simulink Converter8/1 -> Mux2/1
  PS-Simulink Converter10/1 -> Mux2/2
  PS-Simulink Converter12/1 -> Mux2/3
  PS-Simulink Converter9/1 -> Mux3/1
  PS-Simulink Converter11/1 -> Mux3/2
  PS-Simulink Converter13/1 -> Mux3/3
  F/1 -> Saturation3/1
  T/1 -> Demux1/1
  PS-Simulink Converter15/1 -> omega/1, Integrator/1
  MATLAB Function/1(Rout) -> To Workspace2/1, R3x3/1
  Transfer Fcn (with initial outputs)/1 -> Mux4/1, Simulink-PS Converter/1
  Transfer Fcn (with initial outputs)1/1 -> Mux4/2, Simulink-PS Converter2/1
  Transfer Fcn (with initial outputs)2/1 -> Mux4/3, Simulink-PS Converter4/1
  Transfer Fcn (with initial outputs)3/1 -> Mux4/4, Simulink-PS Converter6/1
  Demux1/1 -> Subsystem/1(Td)
  Demux1/2 -> Subsystem1/1(Td)
  Demux1/3 -> Subsystem2/1(Td)
  Demux1/4 -> Subsystem3/1(Td)
  Subsystem/1(Treal) -> Mux5/1, Simulink-PS Converter1/1
  Subsystem1/1(Treal) -> Mux5/2, Simulink-PS Converter3/1
  Subsystem2/1(Treal) -> Mux5/3, Simulink-PS Converter5/1
  Subsystem3/1(Treal) -> Mux5/4, Simulink-PS Converter7/1
  Mux2/1 -> position/1, To Workspace3/1
  Mux3/1 -> acceleration/1
  Demux/1 -> Transfer Fcn (with initial outputs)/1
  Demux/2 -> Transfer Fcn (with initial outputs)1/1
  Demux/3 -> Transfer Fcn (with initial outputs)2/1
  Demux/4 -> Transfer Fcn (with initial outputs)3/1
  Mux4/1 -> To Workspace9/1
  Saturation3/1 -> Demux/1
  Mux5/1 -> To Workspace1/1
  Constant/1 -> Simulink-PS Converter8/1
  Integrator/1 -> To Workspace5/1
  connections:
  Rigid Transform16/LConn1 -- Rigid Transform15/RConn1 -- Solid5/RConn1
  Rigid Transform2/LConn1 -- Rigid Transform1/RConn1
  Rigid Transform14/LConn1 -- Rigid Transform2/RConn1
  Solid4/RConn1 -- External Force and Torque/RConn1 -- Rigid Transform23/RConn1
  Rigid Transform5/LConn1 -- Revolute Joint1/RConn1
  Solid/RConn1 -- Rigid Transform/RConn1
  Revolute Joint5/LConn1 -- Rigid Transform12/RConn1
  Rigid Transform22/LConn1 -- Solid8/RConn1 -- Rigid Transform21/RConn1
  Revolute Joint1/LConn1 -- Rigid Transform4/RConn1
  Mechanism Configuration/RConn1 -- Solid9/RConn1 -- 6-DOF Joint/LConn1 -- World Frame/RConn1 -- Solver Configuration/RConn1
  Solid3/RConn1 -- External Force and Torque3/RConn1 -- Rigid Transform17/RConn1
  Rigid Transform18/LConn1 -- Rigid Transform9/RConn1
  Rigid Transform10/LConn1 -- Rigid Transform18/RConn1
  Revolute Joint6/LConn1 -- Rigid Transform20/RConn1
  Rigid Transform/LConn1 -- Rigid Transform25/RConn1 -- Rigid Transform19/LConn1 -- Rigid Transform9/LConn1 -- Rigid Transform3/LConn1 -- Rigid Transform1/LConn1
  Rigid Transform8/LConn1 -- Rigid Transform3/RConn1
  Simulink-PS Converter/RConn1 -- External Force and Torque/LConn1
  Revolute Joint4/LConn1 -- Rigid Transform16/RConn1
  Solid2/RConn1 -- External Force and Torque2/RConn1 -- Rigid Transform7/RConn1
  Revolute Joint/LConn1 -- Rigid Transform14/RConn1
  Rigid Transform17/LConn1 -- Revolute Joint4/RConn1
  Rigid Transform7/LConn1 -- Revolute Joint2/RConn1
  Simulink-PS Converter1/RConn1 -- External Force and Torque/LConn2
  Rigid Transform6/LConn1 -- Rigid Transform5/RConn1 -- Solid6/RConn1
  Solid1/RConn1 -- External Force and Torque1/RConn1 -- Rigid Transform13/RConn1
  Rigid Transform12/LConn1 -- Rigid Transform11/RConn1 -- Solid7/RConn1
  Rigid Transform20/LConn1 -- Rigid Transform24/RConn1
  Rigid Transform13/LConn1 -- Revolute Joint5/RConn1
  Rigid Transform23/LConn1 -- Revolute Joint7/RConn1
  Rigid Transform11/LConn1 -- Revolute Joint3/RConn1
  Revolute Joint2/LConn1 -- Rigid Transform6/RConn1
  Revolute Joint3/LConn1 -- Rigid Transform10/RConn1
  Revolute Joint7/LConn1 -- Rigid Transform22/RConn1
  Rigid Transform4/LConn1 -- Rigid Transform8/RConn1
  Rigid Transform21/LConn1 -- Revolute Joint6/RConn1
  Rigid Transform24/LConn1 -- Rigid Transform19/RConn1
  Rigid Transform15/LConn1 -- Revolute Joint/RConn1
  PS-Simulink Converter/LConn1 -- Revolute Joint6/RConn2
  Revolute Joint7/RConn2 -- PS-Simulink Converter1/LConn1
  PS-Simulink Converter2/LConn1 -- Revolute Joint3/RConn2
  PS-Simulink Converter3/LConn1 -- Revolute Joint5/RConn2
  PS-Simulink Converter4/LConn1 -- Revolute Joint1/RConn2
  PS-Simulink Converter5/LConn1 -- Revolute Joint2/RConn2
  PS-Simulink Converter6/LConn1 -- Revolute Joint/RConn2
  PS-Simulink Converter7/LConn1 -- Revolute Joint4/RConn2
  Simulink-PS Converter3/RConn1 -- External Force and Torque1/LConn2
  Simulink-PS Converter2/RConn1 -- External Force and Torque1/LConn1
  Simulink-PS Converter5/RConn1 -- External Force and Torque2/LConn2
  Simulink-PS Converter4/RConn1 -- External Force and Torque2/LConn1
  Simulink-PS Converter7/RConn1 -- External Force and Torque3/LConn2
  Simulink-PS Converter6/RConn1 -- External Force and Torque3/LConn1
  PS-Simulink Converter8/LConn1 -- 6-DOF Joint/RConn2
  PS-Simulink Converter9/LConn1 -- 6-DOF Joint/RConn3
  PS-Simulink Converter10/LConn1 -- 6-DOF Joint/RConn4
  PS-Simulink Converter11/LConn1 -- 6-DOF Joint/RConn5
  PS-Simulink Converter12/LConn1 -- 6-DOF Joint/RConn6
  PS-Simulink Converter13/LConn1 -- 6-DOF Joint/RConn7
  PS-Simulink Converter14/LConn1 -- 6-DOF Joint/RConn8
  PS-Simulink Converter15/LConn1 -- 6-DOF Joint/RConn9
  Rigid Transform25/LConn1 -- 6-DOF Joint/RConn1

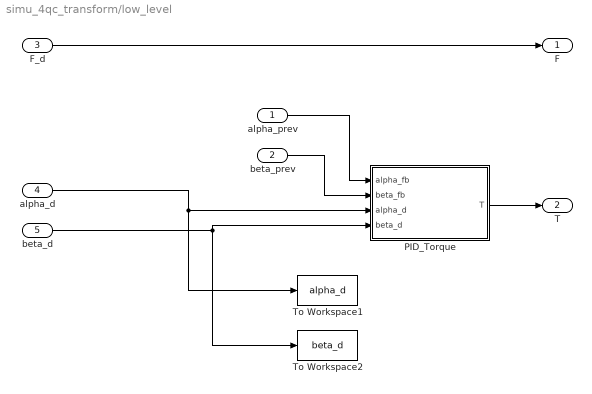
== system simu_4qc_transform/low_level ==
  alpha_prev : Inport
  beta_prev : Inport  Port=2
  F_d : Inport  Port=3
  alpha_d : Inport  Port=4
  beta_d : Inport  Port=5
  PID_Torque : Subsystem
  To Workspace1 : ToWorkspace  VariableName=alpha_d  SaveFormat=Timeseries  SampleTime=-1
  To Workspace2 : ToWorkspace  VariableName=beta_d  SaveFormat=Timeseries  SampleTime=-1
  F : Outport  VectorParamsAs1DForOutWhenUnconnected=off
  T : Outport  Port=2  VectorParamsAs1DForOutWhenUnconnected=off
  wires:
  alpha_prev/1 -> PID_Torque/1(alpha_fb)
  beta_prev/1 -> PID_Torque/2(beta_fb)
  PID_Torque/1(T) -> T/1
  alpha_d/1 -> To Workspace1/1, PID_Torque/3(alpha_d)
  beta_d/1 -> To Workspace2/1, PID_Torque/4(beta_d)
  F_d/1 -> F/1

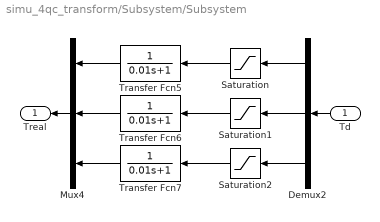
== system simu_4qc_transform/Subsystem/Subsystem ==
  Td : Inport
  Demux2 : Demux  Outputs=3
  Mux4 : Mux  Inputs=3
  Saturation : Saturate  UpperLimit=5.6e-4  LowerLimit=-5.6e-4
  Saturation1 : Saturate  UpperLimit=5.6e-4  LowerLimit=-5.6e-4
  Saturation2 : Saturate  UpperLimit=5.6e-4  LowerLimit=-5.6e-4
  Transfer Fcn5 : TransferFcn  Denominator=[0.01 1]
  Transfer Fcn6 : TransferFcn  Denominator=[0.01 1]
  Transfer Fcn7 : TransferFcn  Denominator=[0.01 1]
  Treal : Outport  VectorParamsAs1DForOutWhenUnconnected=off
  wires:
  Saturation/1 -> Transfer Fcn5/1
  Demux2/1 -> Saturation/1
  Demux2/3 -> Saturation2/1
  Transfer Fcn6/1 -> Mux4/2
  Transfer Fcn5/1 -> Mux4/1
  Saturation1/1 -> Transfer Fcn6/1
  Transfer Fcn7/1 -> Mux4/3
  Demux2/2 -> Saturation1/1
  Saturation2/1 -> Transfer Fcn7/1
  Mux4/1 -> Treal/1
  Td/1 -> Demux2/1

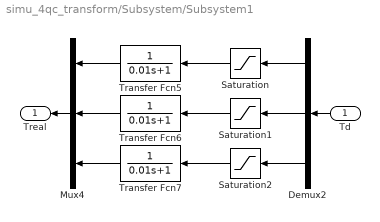
== system simu_4qc_transform/Subsystem/Subsystem1 ==
  Td : Inport
  Demux2 : Demux  Outputs=3
  Mux4 : Mux  Inputs=3
  Saturation : Saturate  UpperLimit=5.6e-4  LowerLimit=-5.6e-4
  Saturation1 : Saturate  UpperLimit=5.6e-4  LowerLimit=-5.6e-4
  Saturation2 : Saturate  UpperLimit=5.6e-4  LowerLimit=-5.6e-4
  Transfer Fcn5 : TransferFcn  Denominator=[0.01 1]
  Transfer Fcn6 : TransferFcn  Denominator=[0.01 1]
  Transfer Fcn7 : TransferFcn  Denominator=[0.01 1]
  Treal : Outport  VectorParamsAs1DForOutWhenUnconnected=off
  wires:
  Saturation/1 -> Transfer Fcn5/1
  Demux2/1 -> Saturation/1
  Demux2/3 -> Saturation2/1
  Transfer Fcn6/1 -> Mux4/2
  Transfer Fcn5/1 -> Mux4/1
  Saturation1/1 -> Transfer Fcn6/1
  Transfer Fcn7/1 -> Mux4/3
  Demux2/2 -> Saturation1/1
  Saturation2/1 -> Transfer Fcn7/1
  Mux4/1 -> Treal/1
  Td/1 -> Demux2/1

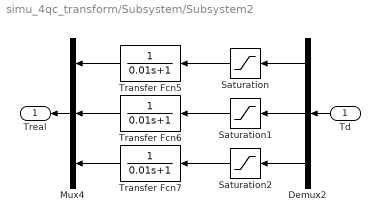
== system simu_4qc_transform/Subsystem/Subsystem2 ==
  Td : Inport
  Demux2 : Demux  Outputs=3
  Mux4 : Mux  Inputs=3
  Saturation : Saturate  UpperLimit=5.6e-4  LowerLimit=-5.6e-4
  Saturation1 : Saturate  UpperLimit=5.6e-4  LowerLimit=-5.6e-4
  Saturation2 : Saturate  UpperLimit=5.6e-4  LowerLimit=-5.6e-4
  Transfer Fcn5 : TransferFcn  Denominator=[0.01 1]
  Transfer Fcn6 : TransferFcn  Denominator=[0.01 1]
  Transfer Fcn7 : TransferFcn  Denominator=[0.01 1]
  Treal : Outport  VectorParamsAs1DForOutWhenUnconnected=off
  wires:
  Saturation/1 -> Transfer Fcn5/1
  Demux2/1 -> Saturation/1
  Demux2/3 -> Saturation2/1
  Transfer Fcn6/1 -> Mux4/2
  Transfer Fcn5/1 -> Mux4/1
  Saturation1/1 -> Transfer Fcn6/1
  Transfer Fcn7/1 -> Mux4/3
  Demux2/2 -> Saturation1/1
  Saturation2/1 -> Transfer Fcn7/1
  Mux4/1 -> Treal/1
  Td/1 -> Demux2/1

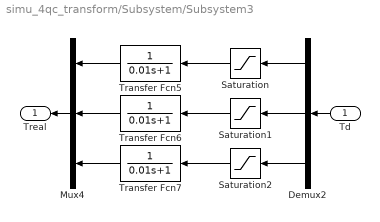
== system simu_4qc_transform/Subsystem/Subsystem3 ==
  Td : Inport
  Demux2 : Demux  Outputs=3
  Mux4 : Mux  Inputs=3
  Saturation : Saturate  UpperLimit=5.6e-4  LowerLimit=-5.6e-4
  Saturation1 : Saturate  UpperLimit=5.6e-4  LowerLimit=-5.6e-4
  Saturation2 : Saturate  UpperLimit=5.6e-4  LowerLimit=-5.6e-4
  Transfer Fcn5 : TransferFcn  Denominator=[0.01 1]
  Transfer Fcn6 : TransferFcn  Denominator=[0.01 1]
  Transfer Fcn7 : TransferFcn  Denominator=[0.01 1]
  Treal : Outport  VectorParamsAs1DForOutWhenUnconnected=off
  wires:
  Saturation/1 -> Transfer Fcn5/1
  Demux2/1 -> Saturation/1
  Demux2/3 -> Saturation2/1
  Transfer Fcn6/1 -> Mux4/2
  Transfer Fcn5/1 -> Mux4/1
  Saturation1/1 -> Transfer Fcn6/1
  Transfer Fcn7/1 -> Mux4/3
  Demux2/2 -> Saturation1/1
  Saturation2/1 -> Transfer Fcn7/1
  Mux4/1 -> Treal/1
  Td/1 -> Demux2/1

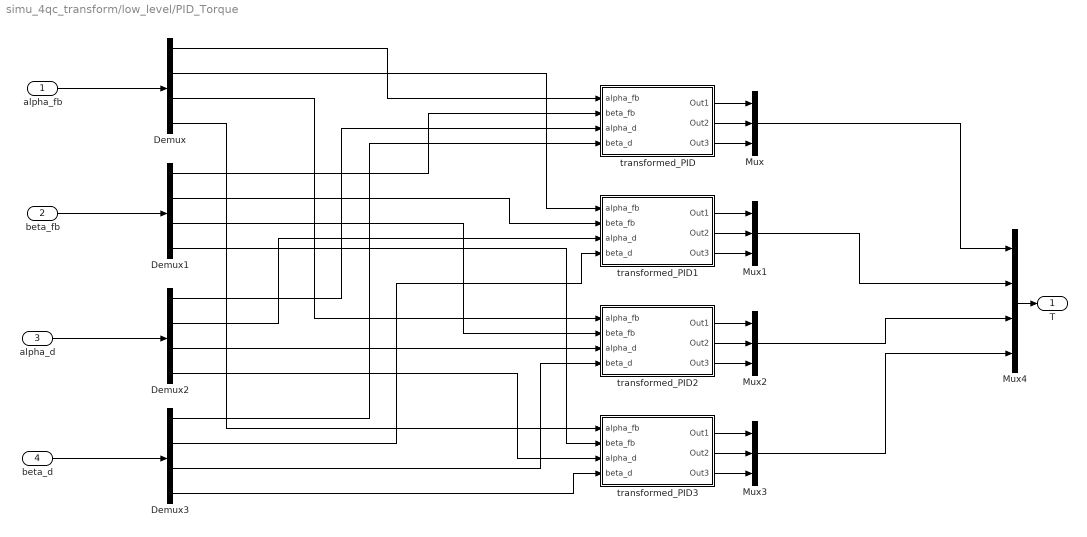
== system simu_4qc_transform/low_level/PID_Torque ==
  alpha_fb : Inport
  beta_fb : Inport  Port=2
  alpha_d : Inport  Port=3
  beta_d : Inport  Port=4
  Demux{,1..3} (4 alike) : Demux
  Mux{,1..3} (4 alike) : Mux  Inputs=3
  Mux4 : Mux
  transformed_PID : Subsystem
  transformed_PID1 : Subsystem
  transformed_PID2 : Subsystem
  transformed_PID3 : Subsystem
  T : Outport  VectorParamsAs1DForOutWhenUnconnected=off
  wires:
  beta_fb/1 -> Demux1/1
  alpha_d/1 -> Demux2/1
  Mux4/1 -> T/1
  Mux/1 -> Mux4/1
  beta_d/1 -> Demux3/1
  alpha_fb/1 -> Demux/1
  transformed_PID/1(Out1) -> Mux/1
  transformed_PID/2(Out2) -> Mux/2
  transformed_PID/3(Out3) -> Mux/3
  transformed_PID1/2(Out2) -> Mux1/2
  transformed_PID1/1(Out1) -> Mux1/1
  transformed_PID1/3(Out3) -> Mux1/3
  transformed_PID2/3(Out3) -> Mux2/3
  transformed_PID2/2(Out2) -> Mux2/2
  transformed_PID3/3(Out3) -> Mux3/3
  transformed_PID3/2(Out2) -> Mux3/2
  Mux1/1 -> Mux4/2
  Mux2/1 -> Mux4/3
  Mux3/1 -> Mux4/4
  transformed_PID2/1(Out1) -> Mux2/1
  transformed_PID3/1(Out1) -> Mux3/1
  Demux/1 -> transformed_PID/1(alpha_fb)
  Demux/2 -> transformed_PID1/1(alpha_fb)
  Demux/3 -> transformed_PID2/1(alpha_fb)
  Demux/4 -> transformed_PID3/1(alpha_fb)
  Demux1/1 -> transformed_PID/2(beta_fb)
  Demux1/2 -> transformed_PID1/2(beta_fb)
  Demux1/3 -> transformed_PID2/2(beta_fb)
  Demux1/4 -> transformed_PID3/2(beta_fb)
  Demux2/1 -> transformed_PID/3(alpha_d)
  Demux2/2 -> transformed_PID1/3(alpha_d)
  Demux2/3 -> transformed_PID2/3(alpha_d)
  Demux2/4 -> transformed_PID3/3(alpha_d)
  Demux3/1 -> transformed_PID/4(beta_d)
  Demux3/2 -> transformed_PID1/4(beta_d)
  Demux3/3 -> transformed_PID2/4(beta_d)
  Demux3/4 -> transformed_PID3/4(beta_d)

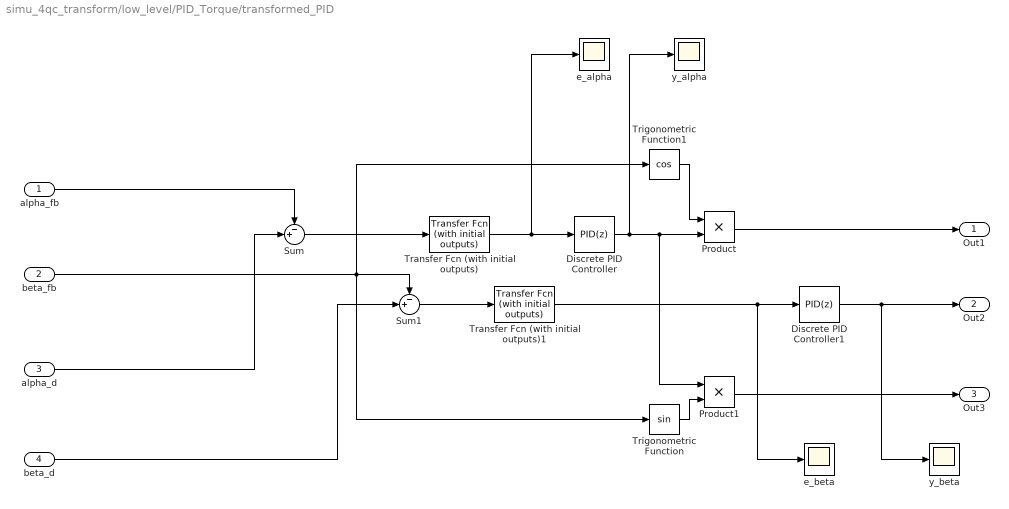
== system simu_4qc_transform/low_level/PID_Torque/transformed_PID ==
  alpha_fb : Inport
  beta_fb : Inport  Port=2
  alpha_d : Inport  Port=3
  beta_d : Inport  Port=4
  Discrete PID Controller : simulink/Continuous/PID Controller  Controller=PID  Form=Parallel  TimeDomain=Discrete-time  UseExternalTs=off  SampleTime=-1  IntegratorMethod=Forward Euler  FilterMethod=Forward Euler  ControllerParametersSource=internal  P=pgaina  I=igaina  D=dgaina  UseFilter=off  N=50  TunerSelectOption=Transfer Function Based (PID Tuner App)  InitialConditionSource=internal  InitialConditionForIntegrator=0  InitialConditionForFilter=0  DifferentiatorICPrevScaledInput=0  ExternalReset=none  TrackingMode=off  Kt=1  LimitOutput=off  UpperSaturationLimit=inf  LowerSaturationLimit=-inf  LinearizeAsGain=off  AntiWindupMode=none  Kb=1  POutMin=[]  POutMax=[]  IOutMin=[]  IOutMax=[]  DOutMin=[]  DOutMax=[]  NOutMin=[]  NOutMax=[]  SumOutMin=[]  SumOutMax=[]  SaturationOutMin=[]  SaturationOutMax=[]  PParamMin=[]  PParamMax=[]  IParamMin=[]  IParamMax=[]  DParamMin=[]  DParamMax=[]  NParamMin=[]  NParamMax=[]  KbParamMin=[]  KbParamMax=[]  KtParamMin=[]  KtParamMax=[]  KbOutMin=[]  KbOutMax=[]  KtOutMin=[]  KtOutMax=[]  IntegratorOutMin=[]  IntegratorOutMax=[]  FilterOutMin=[]  FilterOutMax=[]  SumI1OutMin=[]  SumI1OutMax=[]  SumI2OutMin=[]  SumI2OutMax=[]  SumI3OutMin=[]  SumI3OutMax=[]  SumI4OutMin=[]  SumI4OutMax=[]  SumDOutMin=[]  SumDOutMax=[]  DifferentiatorOutMin=[]  DifferentiatorOutMax=[]  FilterDiffOutCoefMin=[]  FilterDiffOutCoefMax=[]  ReciprocalOutMin=[]  ReciprocalOutMax=[]  SumDenOutMin=[]  SumDenOutMax=[]  SumNumOutMin=[]  SumNumOutMax=[]  DivideOutMin=[]  DivideOutMax=[]  UdiffTsProdOutMin=[]  UdiffTsProdOutMax=[]  NTsProdOutMin=[]  NTsProdOutMax=[]  UintegralTsProdOutMin=[]  UintegralTsProdOutMax=[]  UngainTsProdOutMin=[]  UngainTsProdOutMax=[]  IntegratorContinuousStateAttributes=''  IntegratorStateMustResolveToSignalObject=off  IntegratorRTWStateStorageClass=Auto  FilterContinuousStateAttributes=''  FilterStateMustResolveToSignalObject=off  FilterRTWStateStorageClass=Auto  ParallelPVariant=InternalParameters  IdealPVariant=Disabled  IVariant=InternalParameters  DVariant=InternalParameters  IntegratorVariant=Discrete  SatVariant=Disabled  AWVariant=Passthrough  PCopyVariant=Disabled  TRVariant=Disabled  FdbkBlocksVariant=Forward  IdealPFdbkVariant=Disabled  SatFdbkVariant=Disabled  DerivativeFilterVariant=Differentiator  NVariant=Passthrough  NCopyVariant=Disabled_SignalSpec  FilterICVariant=InternalICsDifferentiator  IntegratorICVariant=InternalICs  ExternalResetVariant=Disabled  TRSumVariant=Passthrough  SumFdbkVariant=Disabled  SumVariant=Sum_PID  TsampFilterVariant=InternalTs  TsampNgainVariant=Passthrough  TsampIntegralVariant=Passthrough
  Discrete PID Controller1 : simulink/Continuous/PID Controller  Controller=PID  Form=Parallel  TimeDomain=Discrete-time  UseExternalTs=off  SampleTime=-1  IntegratorMethod=Forward Euler  FilterMethod=Forward Euler  ControllerParametersSource=internal  P=pgainb  I=igainb  D=dgainb  UseFilter=off  N=50  TunerSelectOption=Transfer Function Based (PID Tuner App)  InitialConditionSource=internal  InitialConditionForIntegrator=0  InitialConditionForFilter=0  DifferentiatorICPrevScaledInput=0  ExternalReset=none  TrackingMode=off  Kt=1  LimitOutput=off  UpperSaturationLimit=inf  LowerSaturationLimit=-inf  LinearizeAsGain=off  AntiWindupMode=none  Kb=1  POutMin=[]  POutMax=[]  IOutMin=[]  IOutMax=[]  DOutMin=[]  DOutMax=[]  NOutMin=[]  NOutMax=[]  SumOutMin=[]  SumOutMax=[]  SaturationOutMin=[]  SaturationOutMax=[]  PParamMin=[]  PParamMax=[]  IParamMin=[]  IParamMax=[]  DParamMin=[]  DParamMax=[]  NParamMin=[]  NParamMax=[]  KbParamMin=[]  KbParamMax=[]  KtParamMin=[]  KtParamMax=[]  KbOutMin=[]  KbOutMax=[]  KtOutMin=[]  KtOutMax=[]  IntegratorOutMin=[]  IntegratorOutMax=[]  FilterOutMin=[]  FilterOutMax=[]  SumI1OutMin=[]  SumI1OutMax=[]  SumI2OutMin=[]  SumI2OutMax=[]  SumI3OutMin=[]  SumI3OutMax=[]  SumI4OutMin=[]  SumI4OutMax=[]  SumDOutMin=[]  SumDOutMax=[]  DifferentiatorOutMin=[]  DifferentiatorOutMax=[]  FilterDiffOutCoefMin=[]  FilterDiffOutCoefMax=[]  ReciprocalOutMin=[]  ReciprocalOutMax=[]  SumDenOutMin=[]  SumDenOutMax=[]  SumNumOutMin=[]  SumNumOutMax=[]  DivideOutMin=[]  DivideOutMax=[]  UdiffTsProdOutMin=[]  UdiffTsProdOutMax=[]  NTsProdOutMin=[]  NTsProdOutMax=[]  UintegralTsProdOutMin=[]  UintegralTsProdOutMax=[]  UngainTsProdOutMin=[]  UngainTsProdOutMax=[]  IntegratorContinuousStateAttributes=''  IntegratorStateMustResolveToSignalObject=off  IntegratorRTWStateStorageClass=Auto  FilterContinuousStateAttributes=''  FilterStateMustResolveToSignalObject=off  FilterRTWStateStorageClass=Auto  ParallelPVariant=InternalParameters  IdealPVariant=Disabled  IVariant=InternalParameters  DVariant=InternalParameters  IntegratorVariant=Discrete  SatVariant=Disabled  AWVariant=Passthrough  PCopyVariant=Disabled  TRVariant=Disabled  FdbkBlocksVariant=Forward  IdealPFdbkVariant=Disabled  SatFdbkVariant=Disabled  DerivativeFilterVariant=Differentiator  NVariant=Passthrough  NCopyVariant=Disabled_SignalSpec  FilterICVariant=InternalICsDifferentiator  IntegratorICVariant=InternalICs  ExternalResetVariant=Disabled  TRSumVariant=Passthrough  SumFdbkVariant=Disabled  SumVariant=Sum_PID  TsampFilterVariant=InternalTs  TsampNgainVariant=Passthrough  TsampIntegralVariant=Passthrough
  Product : Product
  Product1 : Product
  Sum : Sum  Inputs=-+|
  Sum1 : Sum  Inputs=-+|
  Transfer Fcn (with initial outputs) : simulink_extras/Additional Linear/Transfer Fcn (with initial outputs)  N=[1]  D="[0.02  1]"  Y0=0  U0=0
  Transfer Fcn (with initial outputs)1 : simulink_extras/Additional Linear/Transfer Fcn (with initial outputs)  N=[1]  D="[0.02  1]"  Y0=0  U0=0
  Trigonometric Function : Trigonometry  OutputSignalType=real
  Trigonometric Function1 : Trigonometry  Operator=cos  OutputSignalType=real
  e_alpha : Scope
  e_beta : Scope
  y_alpha : Scope
  y_beta : Scope
  Out1 : Outport  VectorParamsAs1DForOutWhenUnconnected=off
  Out2 : Outport  Port=2  VectorParamsAs1DForOutWhenUnconnected=off
  Out3 : Outport  Port=3  VectorParamsAs1DForOutWhenUnconnected=off
  wires:
  Trigonometric Function1/1 -> Product/1
  beta_fb/1 -> Sum1/1, Trigonometric Function1/1, Trigonometric Function/1
  Discrete PID Controller1/1 -> y_beta/1, Out2/1
  Sum1/1 -> Transfer Fcn (with initial outputs)1/1
  alpha_fb/1 -> Sum/1
  alpha_d/1 -> Sum/2
  Sum/1 -> Transfer Fcn (with initial outputs)/1
  Trigonometric Function/1 -> Product1/2
  beta_d/1 -> Sum1/2
  Product1/1 -> Out3/1
  Product/1 -> Out1/1
  Discrete PID Controller/1 -> y_alpha/1, Product1/1, Product/2
  Transfer Fcn (with initial outputs)/1 -> e_alpha/1, Discrete PID Controller/1
  Transfer Fcn (with initial outputs)1/1 -> e_beta/1, Discrete PID Controller1/1
